simulink model "bt2"  (R2021b)
settings: Solver=VariableStepAuto  StartTime=0.0  StopTime=100000  RelTol=1e-3
undefined symbols (not defined in the file): j
libraries: visionstatistics x3, commdigbbndpm3 x2, simulink x2, commsink2 x1, commrandsrc3 x1
settings Model: Creator=Admin  LastModifiedBy=Admin

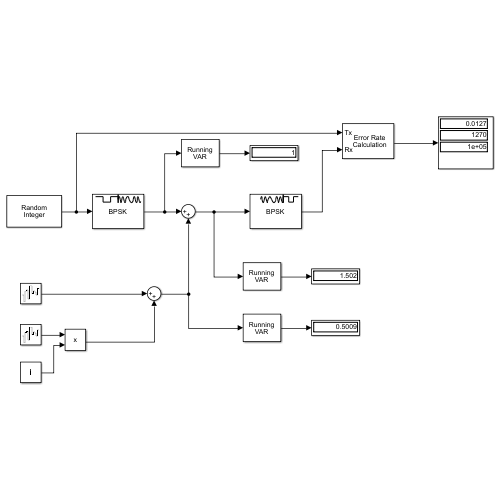
[thumbnail: Simulink's stored preview of the top-level diagram]
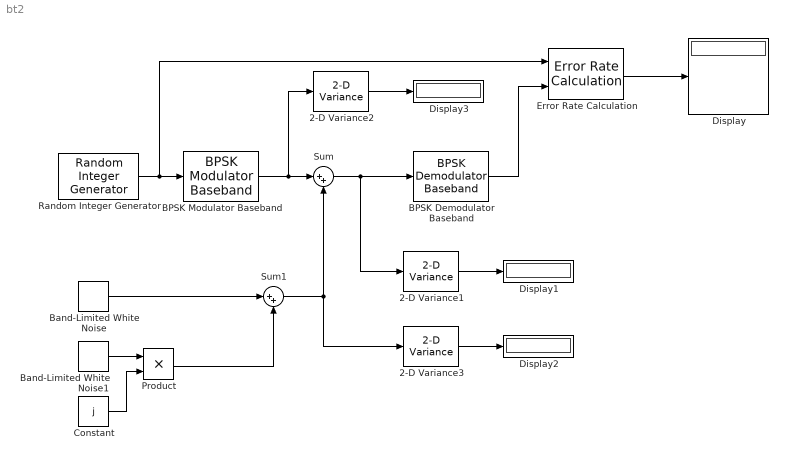
== system bt2 ==
  2-D Variance1 : visionstatistics/2-D Variance  run=on  reset_popup=None  directionMode=Entire input  dimension=1  treatSBRowAsCol=on  roiEnable=off  roiType=Rectangles  roiPortion=Entire ROI  roiOutput=Individual statistics for each ROI  roiFlag=off  roundingMode=Floor  overflowMode=off  prodOutputMode=Binary point scaling  prodOutputWordLength=32  prodOutputFracLength=0  prodOutputSlope=2^0  memorySlope=2^-30  accumSlope=2^-32  outputSlope=2^-32
      settings: SourceProductBaseCode=VP
  2-D Variance2 : visionstatistics/2-D Variance  run=on  reset_popup=None  directionMode=Entire input  dimension=1  treatSBRowAsCol=on  roiEnable=off  roiType=Rectangles  roiPortion=Entire ROI  roiOutput=Individual statistics for each ROI  roiFlag=off  roundingMode=Floor  overflowMode=off  prodOutputMode=Binary point scaling  prodOutputWordLength=32  prodOutputFracLength=0  prodOutputSlope=2^0  memorySlope=2^-30  accumSlope=2^-32  outputSlope=2^-32
      settings: SourceProductBaseCode=VP
  2-D Variance3 : visionstatistics/2-D Variance  run=on  reset_popup=None  directionMode=Entire input  dimension=1  treatSBRowAsCol=on  roiEnable=off  roiType=Rectangles  roiPortion=Entire ROI  roiOutput=Individual statistics for each ROI  roiFlag=off  roundingMode=Floor  overflowMode=off  prodOutputMode=Binary point scaling  prodOutputWordLength=32  prodOutputFracLength=0  prodOutputSlope=2^0  memorySlope=2^-30  accumSlope=2^-32  outputSlope=2^-32
      settings: SourceProductBaseCode=VP
  BPSK Demodulator Baseband : commdigbbndpm3/BPSK Demodulator Baseband  DecType=Hard decision  VarSource=Dialog  Variance=1  Ph=0  outDtype=Inherit via internal rule  derotateFactorWordLen=16  derotateFactorDataTypeStr=Inherit: Same word length as input  derotateFactorLastDataTypeStr=Inherit: Same word length as input
  BPSK Modulator Baseband : commdigbbndpm3/BPSK Modulator Baseband  Ph=0  outDtype=double  outWordLen=16  outUDDataType=sfix(16)  outFracLenMode=Best precision  outFracLen=15  outDataTypeStr=double  outLastDataTypeStr=double
  Band-Limited White Noise : simulink/Sources/Band-Limited White Noise  Cov=[0.19745]  Ts=1  seed=67
  Band-Limited White Noise1 : simulink/Sources/Band-Limited White Noise  Cov=[0.3]  Ts=1  seed=67
  Constant : Constant  Value=j
  Display{,1..3} (4 alike) : Display
  Error Rate Calculation : commsink2/Error Rate Calculation  N=0  st_delay=0  cp_mode=Entire frame  subframe=[]  PMode=Port  WsName=ErrorVec  RsMode2=off  stop=off  numErr=100  maxBits=1e6
  Product : Product
  Random Integer Generator : commrandsrc3/Random Integer Generator  SetSize=2  SeedSource=Parameter  Seed=37  SampleTime=1  SamplesPerFrame=1  OutputDataType=double  SimulateUsing=Interpreted execution
  Sum : Sum  Inputs=|++
  Sum1 : Sum  Inputs=|++
  wires:
  Random Integer Generator/1 -> Error Rate Calculation/1, BPSK Modulator Baseband/1
  BPSK Modulator Baseband/1 -> Sum/1, 2-D Variance2/1
  Error Rate Calculation/1 -> Display/1
  BPSK Demodulator Baseband/1 -> Error Rate Calculation/2
  2-D Variance2/1 -> Display3/1
  Sum/1 -> 2-D Variance1/1, BPSK Demodulator Baseband/1
  Band-Limited White Noise/1 -> Sum1/1
  Constant/1 -> Product/2
  Band-Limited White Noise1/1 -> Product/1
  Product/1 -> Sum1/2
  Sum1/1 -> Sum/2, 2-D Variance3/1
  2-D Variance1/1 -> Display1/1
  2-D Variance3/1 -> Display2/1
